simulink model "Pendulum_Cart_System_Control"  (R2018a)
settings: Solver=VariableStepAuto  StartTime=0.0  StopTime=10.0  RelTol=1e-3
settings Model: Creator=AHMED  LastModifiedBy=AHMED

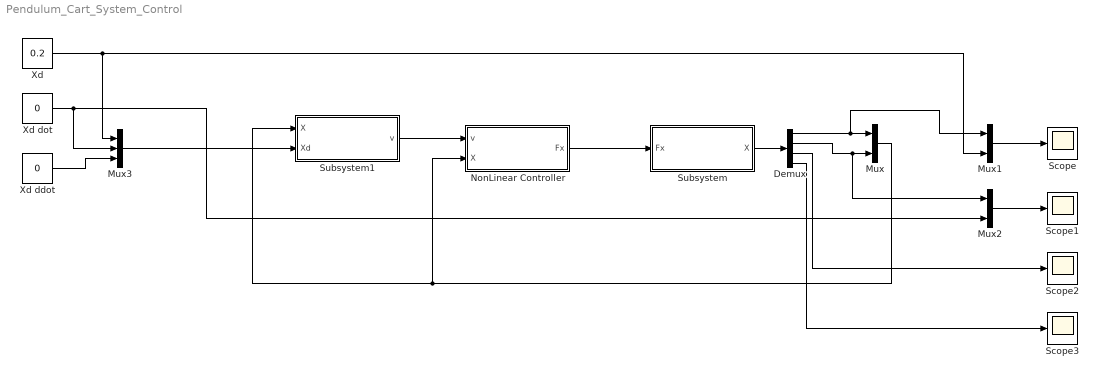
== system Pendulum_Cart_System_Control ==
  Demux : Demux
  Mux : Mux  Inputs=2
  Mux1 : Mux  Inputs=2
  Mux2 : Mux  Inputs=2
  Mux3 : Mux  Inputs=3
  NonLinear Controller : Subsystem
  Scope{,1..3} (4 alike) : Scope
  Subsystem : Subsystem
  Subsystem1 : Subsystem
  Xd : Constant  Value=0.2
  Xd ddot : Constant  Value=0
  Xd dot : Constant  Value=0
  wires:
  NonLinear Controller/1(Fx) -> Subsystem/1(Fx)
  Subsystem1/1(v) -> NonLinear Controller/1(v)
  Mux3/1 -> Subsystem1/2(Xd)
  Subsystem/1(X) -> Demux/1
  Demux/1 -> Mux1/1, Mux/1
  Demux/2 -> Mux2/1, Mux/2
  Mux/1 -> Subsystem1/1(X), NonLinear Controller/2(X)
  Demux/3 -> Scope2/1
  Demux/4 -> Scope3/1
  Mux1/1 -> Scope/1
  Mux2/1 -> Scope1/1
  Xd/1 -> Mux3/1, Mux1/2
  Xd dot/1 -> Mux3/2, Mux2/2
  Xd ddot/1 -> Mux3/3

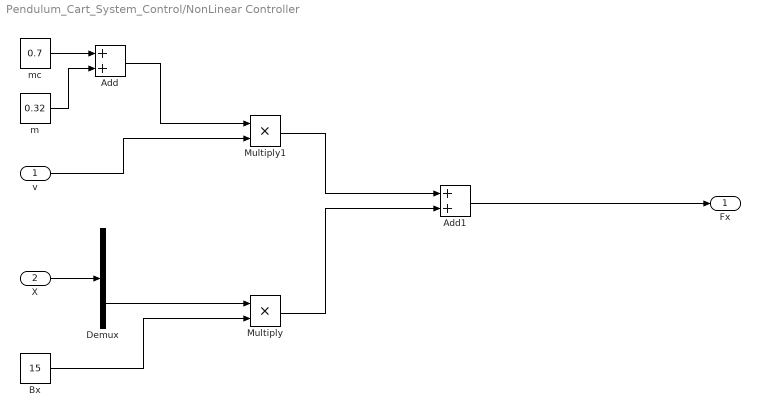
== system Pendulum_Cart_System_Control/NonLinear Controller ==
  v : Inport
  X : Inport  Port=2
  Add : Sum
  Add1 : Sum
  Bx : Constant  Value=15
  Demux : Demux  Outputs=2
  Multiply : Product
  Multiply1 : Product
  m : Constant  Value=0.32
  mc : Constant  Value=0.7
  Fx : Outport
  wires:
  X/1 -> Demux/1
  Demux/2 -> Multiply/1
  Bx/1 -> Multiply/2
  mc/1 -> Add/1
  m/1 -> Add/2
  v/1 -> Multiply1/2
  Add/1 -> Multiply1/1
  Multiply1/1 -> Add1/1
  Multiply/1 -> Add1/2
  Add1/1 -> Fx/1

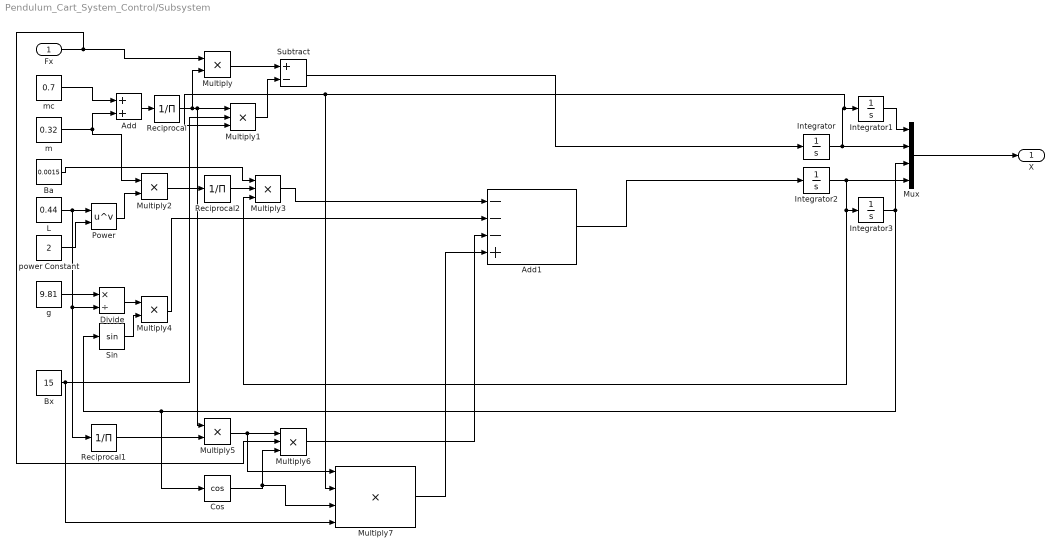
== system Pendulum_Cart_System_Control/Subsystem ==
  Fx : Inport
  Add : Sum
  Add1 : Sum  Inputs=---+
  Ba : Constant  Value=0.0015
  Bx : Constant  Value=15
  Cos : Trigonometry  Operator=cos
  Divide : Product  Inputs=*/
  Integrator{,1..3} (4 alike) : Integrator
  L : Constant  Value=0.44
  Multiply{,2,4..5} (4 alike) : Product
  Multiply1 : Product  Inputs=3
  Multiply3 : Product  Inputs=3
  Multiply6 : Product  Inputs=3
  Multiply7 : Product  Inputs=4
  Mux : Mux
  Power : Math  Operator=pow  SaturateOnIntegerOverflow=on
  Reciprocal : Product  Inputs=/
  Reciprocal1 : Product  Inputs=/
  Reciprocal2 : Product  Inputs=/
  Sin : Trigonometry
  Subtract : Sum  Inputs=+-
  g : Constant  Value=9.81
  m : Constant  Value=0.32
  mc : Constant  Value=0.7
  power Constant : Constant  Value=2
  X : Outport
  wires:
  Mux/1 -> X/1
  Integrator/1 -> Multiply7/2, Multiply1/3, Integrator1/1, Mux/2
  Integrator1/1 -> Mux/1
  Integrator2/1 -> Multiply3/3, Integrator3/1, Mux/4
  Integrator3/1 -> Cos/1, Sin/1, Mux/3
  mc/1 -> Add/1
  m/1 -> Multiply2/1, Add/2
  Multiply/1 -> Subtract/1
  Bx/1 -> Multiply7/4, Multiply1/2
  Multiply1/1 -> Subtract/2
  Add/1 -> Reciprocal/1
  Reciprocal/1 -> Multiply5/1, Multiply1/1, Multiply/2
  Multiply2/1 -> Reciprocal2/1
  L/1 -> Reciprocal1/1, Divide/2, Power/1
  Power/1 -> Multiply2/2
  power Constant/1 -> Power/2
  Reciprocal2/1 -> Multiply3/2
  Ba/1 -> Multiply3/1
  Multiply3/1 -> Add1/1
  Add1/1 -> Integrator2/1
  Subtract/1 -> Integrator/1
  g/1 -> Divide/1
  Divide/1 -> Multiply4/1
  Sin/1 -> Multiply4/2
  Multiply4/1 -> Add1/2
  Reciprocal1/1 -> Multiply5/2
  Multiply5/1 -> Multiply7/1, Multiply6/1
  Fx/1 -> Multiply/1, Multiply6/2
  Cos/1 -> Multiply7/3, Multiply6/3
  Multiply6/1 -> Add1/3
  Multiply7/1 -> Add1/4

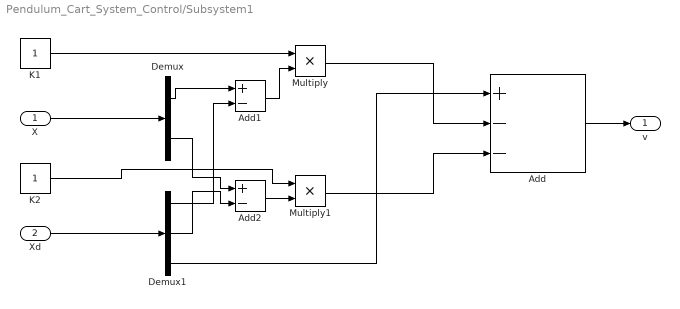
== system Pendulum_Cart_System_Control/Subsystem1 ==
  X : Inport
  Xd : Inport  Port=2
  Add : Sum  Inputs=+--
  Add1 : Sum  Inputs=+-
  Add2 : Sum  Inputs=+-
  Demux : Demux  Outputs=2
  Demux1 : Demux  Outputs=3
  K1 : Constant
  K2 : Constant
  Multiply : Product
  Multiply1 : Product
  v : Outport
  wires:
  X/1 -> Demux/1
  Xd/1 -> Demux1/1
  Add/1 -> v/1
  Demux1/3 -> Add/1
  K1/1 -> Multiply/1
  Add1/1 -> Multiply/2
  Demux/1 -> Add1/1
  Demux1/1 -> Add1/2
  Demux/2 -> Add2/1
  Demux1/2 -> Add2/2
  Add2/1 -> Multiply1/2
  K2/1 -> Multiply1/1
  Multiply/1 -> Add/2
  Multiply1/1 -> Add/3
